simulink model "iv_v_DetectObject"  (R2023a)
settings: Solver=FixedStepDiscrete  StartTime=0.0  StopTime=240  FixedStep=0.01  RelTol=1e-3
undefined symbols (not defined in the file or in its folder): axleLength, DiscIntNeverNeededParam, InputPWM, ticksPerRot, wheelR, WheelSpeed
libraries: mobileRoboticsTrainingLib x7, simulink_extras x2, simulink x1
settings Model: SimulationMode=accelerator  NumberOfSteps=10  SnapshotBufferSize=20  Creator=Boitumelo  LastModifiedBy=cameronclark
settings DebuggingCC: UnconnectedInputMsg=warning  UnconnectedOutputMsg=warning  UnconnectedLineMsg=warning
settings ModelReferenceCC: EnableRefExpFcnMdlSchedulingChecks=on
settings RTWCC: DLArmComputeVersion=19.05

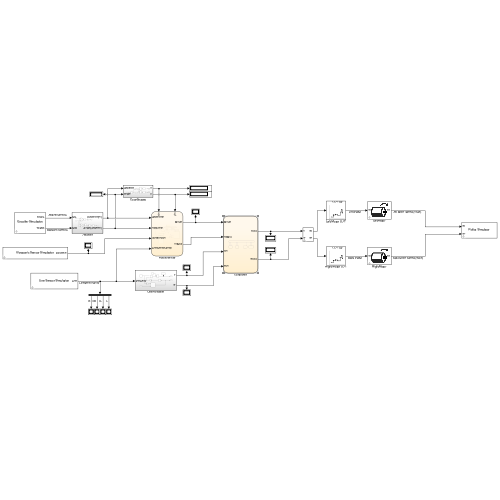
[thumbnail: Simulink's stored preview of the top-level diagram]
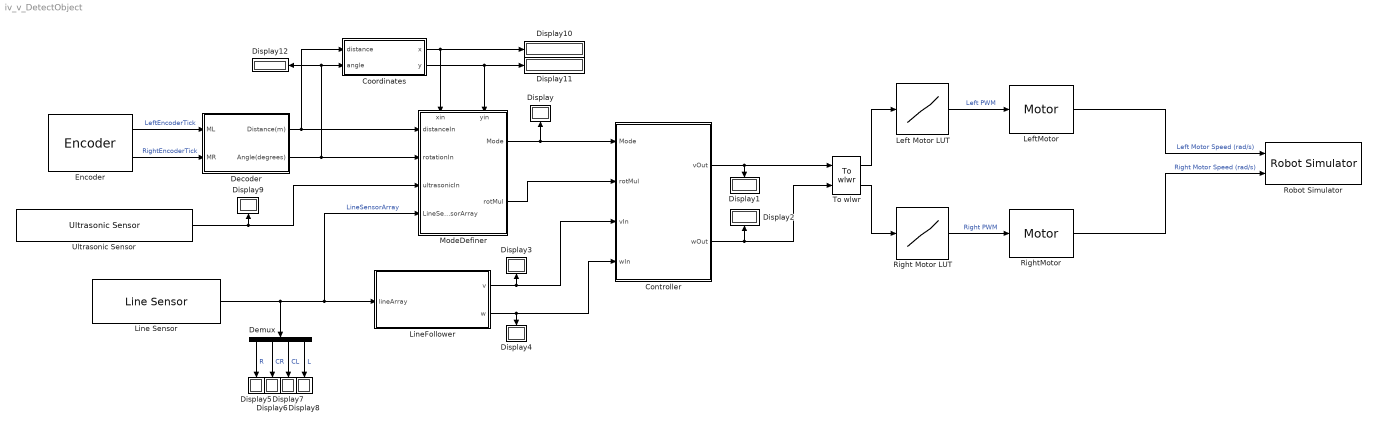
== system iv_v_DetectObject ==
  Controller : Stateflow chart  TreatAsAtomicUnit=on
      settings: PortSchema="{\"entries\":[{\"content\":{\"sides\":[{\"content\":{\"connectorIds\":[\"In2\",\"In1\",\"In3\",\"In4\"]},\"type\":\"ConnectorPlacement.EquallySpacedRectSide\",\"uuid\":\"0e13ea10-b264-4fbc-ab83-bc41241a6c36\"},{\"content\":{\"connectorIds\":[\"Out1\",\"Out2\"],\"side\":\"RIGHT\"},\"type\":\"ConnectorPlacement.EquallySpacedRectSide\",\"uuid\":\"9cddfb1b-e196-4e58-b952-6299e40de404\"},{\"content\":{\"side\":\"TOP\"},\"type\":\"ConnectorPlacement.EquallySpacedRectSide\",\"uuid\":\"e3e699c2-e489-41cc-aace-e70cb50311af\"}]},\"type\":\"ConnectorPlacement.EquallySpacedConnector\",\"uuid\":\"1d087cfb-49f0-41b6-92be-dfee541679f3\"}],\"packageUris\":[\"http://schema.mathworks.com/mf0/Connector/R2020b\"],\"version\":\"1.0\"}"
  Coordinates : Subsystem
  Decoder : Subsystem
  Demux : Demux
  Display{,1..12} (13 alike) : Display
  Encoder : mobileRoboticsTrainingLib/Encoder  axleLength=axleLength  wheelR=wheelR  ticksPerRot=ticksPerRot
      settings: SourceProductName=Mobile Robotics Training Library
  Left Motor LUT : Lookup_n-D  NumberOfTableDimensions=1  BreakpointsForDimension1=WheelSpeed  Table=InputPWM  InterpMethod=Nearest  ExtrapMethod=Clip  InternalRulePriority=Speed  RndMeth=Simplest
  LeftMotor : mobileRoboticsTrainingLib/Motor  motorPlant=wheelMotorModel  sensorType=Speed
      settings: SourceProductName=Mobile Robotics Training Library
  Line Sensor : mobileRoboticsTrainingLib/Line Sensor  mapVariable=mapForSim  envVal=1  lineVal=0  sensOff=[64.3e-3 35.4e-3;67.5e-3 5e-3;67.5e-3 -5e-3;64.3e-3 -35.4e-3]
      settings: SourceProductName=Mobile Robotics Training Library
  LineFollower : Subsystem
  ModeDefiner : Stateflow chart  TreatAsAtomicUnit=on
      settings: PortSchema="{\"entries\":[{\"content\":{\"sides\":[{\"content\":{\"connectorIds\":[\"In4\",\"In5\",\"In3\",\"In6\"]},\"type\":\"ConnectorPlacement.EquallySpacedRectSide\",\"uuid\":\"2e12269d-ccd1-4e68-8415-629d2e368e6d\"},{\"content\":{\"connectorIds\":[\"Out1\",\"Out2\"],\"side\":\"RIGHT\"},\"type\":\"ConnectorPlacement.EquallySpacedRectSide\",\"uuid\":\"1564c0f6-61d7-475f-9f3f-a1f2c1915817\"},{\"content\":{\"connectorIds\":[\"In1\",\"In2\"],\"side\":\"TOP\"},\"type\":\"ConnectorPlacement.EquallySpacedRectSide\",\"uuid\":\"729d5d21-cc85-429f-97c7-0630790832c8\"}]},\"type\":\"ConnectorPlacement.EquallySpacedConnector\",\"uuid\":\"65fad4a7-698e-4a16-b156-07c77b4027bb\"}],\"packageUris\":[\"http://schema.mathworks.com/mf0/Connector/R2020b\"],\"version\":\"1.0\"}"
  Right Motor LUT : Lookup_n-D  NumberOfTableDimensions=1  BreakpointsForDimension1=WheelSpeed  Table=InputPWM  InterpMethod=Nearest  ExtrapMethod=Clip  InternalRulePriority=Speed  RndMeth=Simplest
  RightMotor : mobileRoboticsTrainingLib/Motor  motorPlant=wheelMotorModel  sensorType=Speed
      settings: SourceProductName=Mobile Robotics Training Library
  Robot Simulator : mobileRoboticsTrainingLib/Robot Simulator  Priority=99  mapVar=mapForSim  startX=1  startY=0.27175  startTheta=90  axleLength=axleLength  wheelR=wheelR
  To wlwr : mobileRoboticsTrainingLib/To wlwr  axleLength=0.1  wheelR=0.05
      link override change parameters: Gain=[1 -axleLength/2;1 axleLength/2]
  Ultrasonic Sensor : mobileRoboticsTrainingLib/Ultrasonic Sensor  mapVar=mapForSim  maxSenRange=2  minSenRange=0.02  senRes=0.01  sensOff=[0 0]
      settings: SourceProductName=Mobile Robotics Training Library
  wires:
  Right Motor LUT/1 -> RightMotor/1  "Right PWM"
  Left Motor LUT/1 -> LeftMotor/1  "Left PWM"
  Encoder/1 -> Decoder/1(ML)  "LeftEncoderTick"
  Encoder/2 -> Decoder/2(MR)  "RightEncoderTick"
  To wlwr/1 -> Left Motor LUT/1
  To wlwr/2 -> Right Motor LUT/1
  RightMotor/1 -> Robot Simulator/2  "Right Motor Speed (rad/s)"
  LeftMotor/1 -> Robot Simulator/1  "Left Motor Speed (rad/s)"
  Line Sensor/1 -> Demux/1, ModeDefiner/6(LineSensorArray), LineFollower/1(lineArray)  "LineSensorArray"
  LineFollower/2(w) -> Display4/1, Controller/4(wIn)
  Controller/1(vOut) -> To wlwr/1, Display1/1
  Controller/2(wOut) -> Display2/1, To wlwr/2
  LineFollower/1(v) -> Display3/1, Controller/3(vIn)
  Demux/1 -> Display5/1  "R"
  Demux/2 -> Display6/1  "CR"
  Demux/4 -> Display8/1  "L"
  Demux/3 -> Display7/1  "CL"
  Ultrasonic Sensor/1 -> Display9/1, ModeDefiner/3(ultrasonicIn)
  ModeDefiner/1(Mode) -> Display/1, Controller/2(Mode)
  ModeDefiner/2(rotMul) -> Controller/1(rotMul)
  Decoder/1(Distance(m)) -> Coordinates/1(distance), ModeDefiner/4(distanceIn)
  Decoder/2(Angle(degrees)) -> Coordinates/2(angle), Display12/1, ModeDefiner/5(rotationIn)
  Coordinates/1(x) -> Display10/1, ModeDefiner/1(xin)
  Coordinates/2(y) -> Display11/1, ModeDefiner/2(yin)

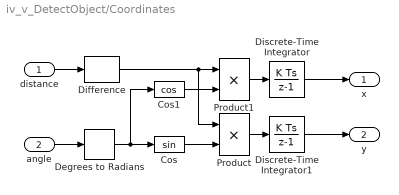
== system iv_v_DetectObject/Coordinates ==
  distance : Inport
  angle : Inport  Port=2
  Cos : Trigonometry
  Cos1 : Trigonometry  Operator=cos
  Degrees to Radians : simulink_extras/Transformations/Degrees to Radians
  Difference : simulink/Discrete/Difference  ICPrevInput=0.0  InputProcessing=Columns as channels (frame based)  OutMin=[]  OutMax=[]  OutDataType=fixdt(1, 16)  OutScaling=2^-10  DoSatur=off
  Discrete-Time Integrator : DiscreteIntegrator  gainval=100  SampleTime=-1  ICPrevOutput=DiscIntNeverNeededParam  ICPrevScaledInput=DiscIntNeverNeededParam
  Discrete-Time Integrator1 : DiscreteIntegrator  gainval=100  SampleTime=-1  ICPrevOutput=DiscIntNeverNeededParam  ICPrevScaledInput=DiscIntNeverNeededParam
  Product : Product
  Product1 : Product
  x : Outport
  y : Outport  Port=2
  wires:
  distance/1 -> Difference/1
  Difference/1 -> Product1/1, Product/1
  Product/1 -> Discrete-Time Integrator1/1
  Product1/1 -> Discrete-Time Integrator/1
  angle/1 -> Degrees to Radians/1
  Degrees to Radians/1 -> Cos1/1, Cos/1
  Cos/1 -> Product/2
  Cos1/1 -> Product1/2
  Discrete-Time Integrator/1 -> x/1
  Discrete-Time Integrator1/1 -> y/1

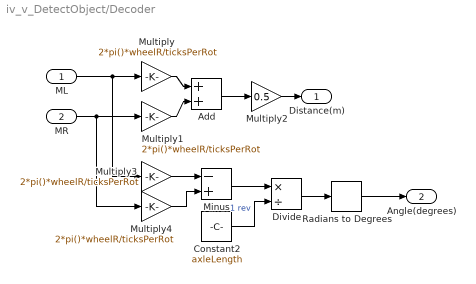
== system iv_v_DetectObject/Decoder ==
  ML : Inport
  MR : Inport  Port=2
  Add : Sum
  Constant2 : Constant  Value=axleLength
  Divide : Product  Inputs=*/
  Minus : Sum  Inputs=-+
  Multiply{,1,3..4} (4 alike) : Gain  Gain=2*pi()*wheelR/ticksPerRot
  Multiply2 : Gain  Gain=0.5
  Radians to Degrees : simulink_extras/Transformations/Radians to Degrees
  Distance(m) : Outport
  Angle(degrees) : Outport  Port=2
  wires:
  Add/1 -> Multiply2/1
  Multiply1/1 -> Add/2
  Multiply/1 -> Add/1
  Multiply2/1 -> Distance(m)/1
  MR/1 -> Multiply1/1, Multiply4/1
  ML/1 -> Multiply3/1, Multiply/1
  Constant2/1 -> Divide/2  "1 rev"
  Divide/1 -> Radians to Degrees/1
  Minus/1 -> Divide/1
  Multiply3/1 -> Minus/1
  Multiply4/1 -> Minus/2
  Radians to Degrees/1 -> Angle(degrees)/1

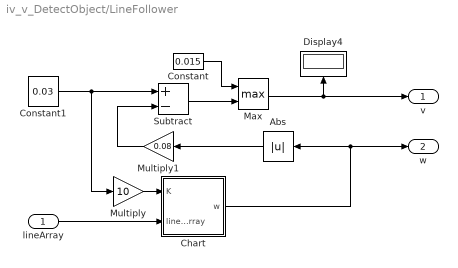
== system iv_v_DetectObject/LineFollower ==
  lineArray : Inport
  Abs : Abs  SaturateOnIntegerOverflow=off
  Chart : Stateflow chart  TreatAsAtomicUnit=on
  Constant : Constant  Value=0.015
  Constant1 : Constant  Value=0.03
  Display4 : Display
  Max : MinMax  Function=max  Inputs=2
  Multiply : Gain  Gain=10
  Multiply1 : Gain  Gain=0.08
  Subtract : Sum  Inputs=+-
  v : Outport
  w : Outport  Port=2
  wires:
  Multiply/1 -> Chart/1(K)
  Constant1/1 -> Subtract/1, Multiply/1
  Subtract/1 -> Max/2
  Multiply1/1 -> Subtract/2
  Abs/1 -> Multiply1/1
  Max/1 -> v/1, Display4/1
  Constant/1 -> Max/1
  lineArray/1 -> Chart/2(lineArray)
  Chart/1(w) -> w/1, Abs/1

== stateflow chart iv_v_DetectObject/ModeDefiner ==
  state Start
    entry:
    Mode = 0;
    intersections = -1 * ones(5,3,4) %[x y;angle1-4;visited1-4]
    intersection = 1;
    currentIntersection = 1;
    objects = -1 * ones(5, 3); %[x y distance rotation]
    object = 1;
    stopZoneFound = 0;
    defaultPath=2
  state RotateBackToLine
    entry:
    Mode = 4;
    rotMul = rotMul * -1;
    exit:
    Mode = 0;
  state ExploreMode
  state RotateToLine
    entry:
    if (LineSensorArray(1) == 0)
    rotMul = 1;
    else
    rotMul = -1;
    end
    Mode = 4;
  state DriveBackToLine
    entry:
    Mode = 0;
    distanceTarget = distanceIn + 60e-3
  state DriveOffStopZone
    entry:
    Mode = 0;
    distanceTarget = distanceIn + 40e-3
  state DriveToUltrasonicLine
    entry:
    Mode = 0;
    distanceTarget = distanceIn + 60e-3
  state DriveOffIntersection
    entry:
    Mode = 0;
    distanceTarget = distanceIn + 40e-3;
  state TurnAround
    entry:
    Mode = 4;
    rotationTarget = rotationIn + 180;
    rotMul = 1;
  state RecordObject
    entry:
    objects(object,:) = [xin yin ultrasonicIn rotationIn];
    object = object + 1;
  state CentreOnIntersection
    entry:
    if (LineSensorArray(1) == 0)
    rotMul = 1;
    else
    rotMul = -1;
    end
    distanceTarget = distanceIn + 60e-3;
  state PickIntersection
    entry:
    display(defaultPath)
    display(intersections)
    Mode = 4;
    if stopZoneFound
    if ~any(intersections(currentIntersection,3,:)==3)
    for path = 1:4
    if abs(abs(mod(intersections(currentIntersection,2,path)-rotationIn,360))-180) <= 25
    intersections(currentIntersection,3,path) = 3;
    break;
    end
    end
    end
    end
    if any(intersections(currentIntersection,3,:)==0)
    %there is an unexplored path
    for path = 4:-1:1
    if ~intersections(currentIntersection,3,path)
    intersections(currentIntersection,3,path) = 1;
    rotationTarget = intersections(currentIntersection,2,path)
    if rotationTarget-rotationIn > 0
    rotMul = 1;
    else
    rotMul = -1;
    end
    break;
    end
    end
    else
    %go back down return path
    for path = 1:4
    if intersections(currentIntersection,3,path)==defaultPath
    rotationTarget = intersections(currentIntersection,2,path)
    if rotationTarget-rotationIn > 0
    rotMul = 1;
    else
    rotMul = -1;
    end
    break
    end
    end
    end
    exit:
    display(defaultPath)
    display(intersections)
  state Stop
    entry:
    Mode = 3;
    display(objects)
  state CheckForOldIntersection
    entry:
    oldIntersection = 0;
    for currentIntersection = 1:5
    if ~all(intersections(currentIntersection,3,:)==-1)
    if abs(intersections(currentIntersection,1,1)-xin) <= 0.1
    if abs(intersections(currentIntersection,1,2)-yin) <= 0.1
    oldIntersection = 1;
    break;
    end
    end
    end
    end
  state SenseNewIntersection
    entry:
    Mode = 4;
    if all(LineSensorArray(2:3)==0)
    rotationTarget = 0;
    else
    rotationTarget = rotationIn + 45*rotMul;
    end
    rotationHalf = rotationIn + 180*rotMul;
    rotationFull = rotationIn + 360*rotMul;
    lineSensorRising = 2.5 - 0.5*rotMul;
    lineSensorFalling = 2.5 + 0.5*rotMul;
    risingEdge = LineSensorArray(lineSensorRising);
    fallingEdge = LineSensorArray(lineSensorFalling);
    fallingEdgeDetected = 0;
    rotationFalling = 0;
    path = 1;
    if (~LineSensorArray(2) | ~LineSensorArray(3))
    %robot is facing an intersection
    intersections(intersection,2,path) = rotationIn;
    intersections(intersection,3,path) = 0;
    path = path + 1;
    end
    during:
    if rotationTarget
    if (rotMul*(rotationTarget-rotationIn) >= 0) & all(LineSensorArray(2:3)==0)
    Mode = 1;
    end
    end
    if fallingEdge & ~LineSensorArray(lineSensorFalling)
    rotationFalling = rotationIn;
    fallingEdgeDetected = 1;
    end
    if ~risingEdge & LineSensorArray(lineSensorRising)
    if fallingEdgeDetected
    intersections(intersection,2,path) = round((rotationIn + rotationFalling)/2/90)*90;
    fallingEdgeDetected = 0;
    if rotationHalf & (abs(intersections(intersection,2,path) - rotationHalf) <= 30)
    %path we came from, thus visited=true
    intersections(intersection,3,path) = 2 + stopZoneFound;
    rotationHalf = 0;
    else
    intersections(intersection,3,path) = 0;
    end
    path = path + 1;
    end
    end
    risingEdge = LineSensorArray(lineSensorRising);
    fallingEdge = LineSensorArray(lineSensorFalling);
  state AddIntersection
    entry:
    %next intersection in array
    intersections(intersection,1,1) = xin;
    intersections(intersection,1, 2) = yin;
    currentIntersection = intersection;
    intersection = intersection + 1;
  (default) -> Start
  Start -> ExploreMode
  DriveBackToLine -> RotateBackToLine : [distanceIn>=distanceTarget]
  RotateBackToLine -> ExploreMode : [all(LineSensorArray(2:3)==0)]
  ExploreMode -> (junction 118) [order 1] : [(LineSensorArray(1) == 0) | (LineSensorArray(4) == 0)]
  ExploreMode -> TurnAround [order 2] : [all(LineSensorArray==1)]
  DriveOffStopZone -> ExploreMode : [distanceIn >= distanceTarget]
  DriveOffIntersection -> ExploreMode : [distanceIn >= distanceTarget]
  RotateToLine -> DriveBackToLine : [all(LineSensorArray(2:3)==0)]
  (junction 118) -> RotateToLine [order 2] : [all(LineSensorArray(2:3)==1)]
  (junction 118) -> DriveToUltrasonicLine [order 1] : [ultrasonicIn & (ultrasonicIn <= 0.5)]
  (junction 118) -> CentreOnIntersection [order 3]
  SenseNewIntersection -> DriveBackToLine [order 1] : [Mode==1]
  DriveToUltrasonicLine -> RecordObject : [distanceIn>=distanceTarget]
  TurnAround -> DriveOffStopZone : [rotationIn>rotationTarget]
  RecordObject -> TurnAround
  PickIntersection -> DriveOffIntersection : [rotMul*(rotationTarget-rotationIn) <= 0]
  (junction 99) -> TurnAround [order 1] : [any(any(intersections(:,3,:) == 0))]{stopZoneFound =1;}
  CentreOnIntersection -> (junction 93) : [distanceIn >= distanceTarget]
  (junction 93) -> (junction 99) [order 1] : [all(LineSensorArray==0)]
  (junction 93) -> CheckForOldIntersection [order 2]
  (junction 99) -> Stop [order 2]
  CheckForOldIntersection -> (junction 113) [order 2] : [oldIntersection]
  (junction 113) -> PickIntersection [order 1] : [any(any(intersections(:,3,:)==0))]{defaultPath=2;}
  (junction 113) -> PickIntersection [order 2] : {defaultPath=3;}
  CheckForOldIntersection -> SenseNewIntersection [order 1] : [~oldIntersection]
  AddIntersection -> PickIntersection
  SenseNewIntersection -> AddIntersection [order 2] : [~rotationHalf & (abs(rotationIn - rotationFull) <= 10)]{defaultPath==2}
  data: xin input; yin input; ultrasonicIn input; Mode output =0; rotMul output; distanceIn input; distanceTarget local; rotationIn input; LineSensorArray input; fallingEdge local; rotationHalf local; rotationFull local; intersection local; path local; rotationTarget local; risingEdge local; lineSensorFalling local; lineSensorRising local; rotationFalling local; fallingEdgeDetected local; intersections local; oldIntersection local; currentIntersection local; stopZoneFound local; defaultPath local; object local; objects local

== stateflow chart iv_v_DetectObject/Controller ==
  state StartBlock
  state Rotate
    during:
    wOut = 0.51*rotMul;
    vOut = 0;
  state Drive
    during:
    wOut = wIn;
    vOut = vIn;
  state DriveForward
    entry:
    wOut = 0;
    vOut = 0.03;
  state Stop
    en:
    vOut=0;
    wOut=0;
  Drive -> StartBlock : [Mode~=0]
  StartBlock -> Drive [order 1] : [Mode==0]
  DriveForward -> StartBlock : [Mode~=1]
  StartBlock -> DriveForward [order 4] : [Mode==1]
  StartBlock -> Stop [order 3] : [Mode==3]
  Rotate -> StartBlock : [Mode~=4]
  StartBlock -> Rotate [order 2] : [Mode==4]
  (default) -> Drive
  data: rotMul input; Mode input; vIn input; wIn input; vOut output; wOut output

== stateflow chart iv_v_DetectObject/LineFollower/Chart ==
  state ComputeW
    %code for the line array
    during:
    w = K*(lineArray(3)-lineArray(2));
  (default) -> ComputeW
  data: w output; K input; lineArray input
